simulink model "EcoSIM3_P2_C2_WIP"  (R2014b)
settings: Solver=ode1  SolverMode=SingleTasking  StartTime=0.0  StopTime=inf  FixedStep=0.01  RelTol=1e-3
PostLoadFcn:
  | %, if any(exist('dsrtsu_mdlpostloadfcn', 'file') == [2, 3, 6]), try dsrtsu_mdlpostloadfcn('Execute', bdroot); catch fprintf('Error in PostLoadFcn (dsrtsu_mdlpostloadfcn) for model "%s":\n %s\n', bdroot, lasterr); end, end,
InitFcn:
  | tic
  | %Startup_EcoSIM
values from neighbouring files (symbols this model uses):
  EngPwr = [0 5	10	15	20	25	30	35	40	45	50	55	60	65	70	75	80	85	90	95	100	105	110	115]    [Series_Maps.m]
  EngSpd = [0 477.4645 954.929 1909.858 2864.787 3819.716 4774.645 5729.574 6684.503]    [Series_Maps.m]
  EngTrq = [0	0	0	0	0	0	0	0	0	0	0	0	0	0	0	0	0	0	0	0	0	0	0	0 ... (first row only)    [Series_Maps.m]
  Power = [0 5 10 15 20 25 30]    [Series_Maps.m]
  Torque = [-50,-40,-30,-25,-20,-15,-10,-8,-6,-4,-2,0]    [Series_Maps.m]
undefined symbols (not defined in the file or in its folder): canChannel, Controls, DriveCycles, Driver, EM_EFF_MAP, EM_PwrLoss_MAP, Glbl, Overwritten_Mode, Plants, sigbuilder_block, Trialmap, Veh_Dynamics
libraries: simulink x141, canmsglib x113, fl_lib x104, canlib x89, nesl_utility x56, sdl_lib x29, dspsigops x6, dspswit3 x5, dspstat3 x2, commnoisgen2 x1, dspfdesign x1
(part 20 of 21)

== stateflow chart EcoSIM3_P2_C2_WIP/Powertrain/Electric Motor /Soft ECU/Algorithm/Startup_Shutdown/Startup-Shutdown ==
  state StartupShutdownSequence [group]
    state StartState
      entry: VSM_Mode = 0;
      during: Commanded_Torque = 0;
      %Loading EEPROM Parameters & carrying out POST (Power On Self Tests)
    state Standby
      % Entry point into Inverter
      % State Machine
    state Startup_Sequence
      state Inverter_Wait
        entry: VSM_Mode = 4;
        during: VSM_Mode = 4;
        during: Commanded_Torque =0;
        % Precharge_Bypasseed_EEPROM = 1
      state ReadyState
        entry: VSM_Mode = 5;
        during: VSM_Mode = 5;
        during: Commanded_Torque =0;
        en, du: Inverter_Enable_Lockout = 0;
      state MotorRunningState
        entry: Inverter_Enable_Lockout = 0;
        entry: Inverter_Status=1;
        during: Inverter_Enable_Lockout = 0;
      state MotorOnCommand
        entry: VSM_Mode=6;
      Inverter_Wait -> ReadyState : [KeySwMode == 0 && ...
          | Power_up==1]
      MotorOnCommand -> ReadyState [order 3] : [Inverter_Enable==0]
      ReadyState -> MotorRunningState : after(0.05,sec)
      MotorRunningState -> MotorOnCommand : [InternalMotorError==0 && Inverter_Enable == 1]
    state ShutdownInProcess
      entry: VSM_Mode = 14;
      entry: Inverter_Enable_Lockout=1;
      entry: Inverter_Status=0;
      during: VSM_Mode = 14;
    state FaultState
      entry: VSM_Mode = 7;
      during: VSM_Mode = 7;
    (junction 28) -> Standby [order 2]
    Standby -> StartState : [Power_up == 1]
    (default) -> (junction 28)
    ShutdownInProcess -> Standby : [KeySwMode == 0 && ...
        | Power_up == 0]
    StartState -> FaultState [order 2] : [POST_Fault == 1]
    StartState -> Inverter_Wait [order 1] : [Power_up ==1 && ...
        | ~InternalMotorError && POST_Fault == 0 ...
        | && batt_mainc_stat == 1 ]
    (junction 28) -> FaultState [order 1] : [InternalMotorError ==1]
    FaultState -> ShutdownInProcess : [(KeySwMode == 0 && ...
        | Power_up == 0) ]
    MotorOnCommand -> ShutdownInProcess [order 1] : [ShutdownRequest ==1]
    MotorOnCommand -> FaultState [order 2] : [RUN_Fault==1]
  data: Power_up input; VSM_Mode output; InternalMotorError input; batt_mainc_stat input; Inverter_Enable input; Inverter_Enable_Lockout output; RUN_Fault input; Commanded_Torque local; ShutdownRequest input; KeySwMode input; POST_Fault input; Inverter_Status output

== stateflow chart EcoSIM3_P2_C2_WIP/Powertrain/Electric Motor /Soft ECU/Algorithm/Normal Operation/Normal_Operation ==
  state NormalOperation
    entry: set_direction=Rotation_Direction;
    entry: ShutdownRequest=0;
    exit: Commanded_Torque=0;
    state SpeedGreaterThanMaxSpeed
      entry: Commanded_Torque=0;
    state ValidSpeed
      entry: Commanded_Torque=Torque_Command;
      during: Commanded_Torque=Torque_Command;
    (default) -> (junction 9)
    (junction 9) -> SpeedGreaterThanMaxSpeed [order 1] : [abs (Motor_Speed) > Motor_MaxSpeed]
    (junction 9) -> (junction 10) [order 2]
    SpeedGreaterThanMaxSpeed -> (junction 10) : [abs (Motor_Speed) <= Motor_MaxSpeed]
    (junction 10) -> ValidSpeed
    ValidSpeed -> SpeedGreaterThanMaxSpeed : [abs (Motor_Speed) > Motor_MaxSpeed]
  state Fault
    entry: RUN_Fault=1;
  state ShutdownRequest
    entry: ShutdownRequest=1;
  (default) -> NormalOperation
  NormalOperation -> Fault [order 1] : [ InternalMotorError ==1||batt_mainc_stat==0]
  NormalOperation -> ShutdownRequest [order 2] : [Power_up==0]
  ShutdownRequest -> NormalOperation : [Power_up==1]
  data: Motor_Speed input; InternalMotorError input; Rotation_Direction input; set_direction local; Commanded_Torque output; Torque_Command input; batt_mainc_stat input; Inverter_Enable input; Power_up input; RUN_Fault output; Motor_MaxSpeed input; ShutdownRequest output

== stateflow chart EcoSIM3_P2_C2_WIP/GCM/ProcessMode/Chart ==
  state Entry
    entry: charge_mode_request=0;
    Relay_Charge=0;
    Relay_Vehicle=0;
  state FaultMode
  state VehicleRunMode
    entry: charge_mode_request=0;
    Relay_Charge=1;
    Relay_Vehicle=1;
  state ChargingMode
    entry: charge_mode_request=1;
    Relay_Charge=1;
    Relay_Vehicle=0;
  (default) -> Entry
  VehicleRunMode -> Entry : [Key_State==0]
  ChargingMode -> Entry [order 1] : [GCM_Wakeup_charge==0]
  Entry -> VehicleRunMode [order 1] : [Key_State==1 && ...
      | GCM_Wakeup_charge==0]
  Entry -> FaultMode [order 3] : [Key_State==1 && ...
      | GCM_Wakeup_charge ==1]
  Entry -> ChargingMode [order 2] : [Key_State ==0 && ...
      | GCM_Wakeup_charge==1]
  ChargingMode -> FaultMode [order 2] : [Key_State==1]
  data: Key_State input; GCM_Wakeup_charge input; Relay_Charge output; Relay_Vehicle output; charge_mode_request output

== matlab function EcoSIM3_P2_C2_WIP/Supervisory Controller/Functional Safety1/Functional Safety Algorithm/Fault Management/Truth Table ==
  data: u input; y output
function y = fcn(u)

aVarTruthTableCondition_1 = false;
aVarTruthTableCondition_2 = false;


% Example condition 1

aVarTruthTableCondition_1 = logical(u >= 0);

% Example condition 2

aVarTruthTableCondition_2 = logical(u ^ 2 <= 1);

if (aVarTruthTableCondition_1 && aVarTruthTableCondition_2)
    aFcnTruthTableAction_1();
elseif (~aVarTruthTableCondition_1 && ~aVarTruthTableCondition_2)
    aFcnTruthTableAction_1();
else % Default
    aFcnTruthTableAction_2();
end

function aFcnTruthTableAction_1()

% Example action 1 called from D1 & D2 column in condition table

y = u;

function aFcnTruthTableAction_2()

% Example action 2 called from D3 column in condition table

y = 1 / u;

== stateflow chart EcoSIM3_P2_C2_WIP/Powertrain/Clutch_Transmission1/CP1 SoftEcu/Algorithm/Chart ==
  note: Clutch_Sw - 0= Clutch fully engaged
      |                        1= Clutch fully disengaged (Pedal completely pressed
      |                        2= Engagement/ Disengagement in process (This state has been introduced so that Mastershift does not shift
      | accidentally while clutch is being engaged, and GCM does not allow torque transmission before clutch is fully engaged
      |
      | Clutch_Request- Request to press (disengage) the clutch
      | 0= Engage the clutch  (Foot off the pedal)
      | 1= Disengage the clutch (Press the pedal)
  state Default
  state DisengageClutch
    entry: Clutch_Engage=0;
    entry: Clutch_Sw=2;
    during: Clutch_Sw=2;
  state ClutchDisengaged
    entry: Clutch_Engage=0;
    entry:Clutch_Sw=1;
  state EngageClutch
    entry: Clutch_Engage=1;
    entry: Clutch_Sw=2;
    during: Clutch_Sw=2;
  state ClutchEngaged
    entry: Clutch_Engage=1;
    entry:Clutch_Sw=0;
    during:Clutch_Sw=0;
  (default) -> Default
  Default -> EngageClutch [order 2] : [Clutch_Request==0]
  Default -> DisengageClutch [order 1] : [Clutch_Request==1]
  ClutchEngaged -> DisengageClutch : [Clutch_Request==1]
  DisengageClutch -> ClutchDisengaged [order 2] : [Clutch_Pressure<=5]
  EngageClutch -> DisengageClutch [order 2] : [Clutch_Request==1]
  DisengageClutch -> EngageClutch [order 1] : [Clutch_Request==0]
  ClutchDisengaged -> EngageClutch : [Clutch_Request==0]
  EngageClutch -> ClutchEngaged [order 1] : [Clutch_Pressure>=10]
  data: Clutch_Request input; Clutch_Pressure input; Clutch_Engage output; Clutch_Sw output

== stateflow chart EcoSIM3_P2_C2_WIP/Supervisory Controller/Mode Operation/Limited EV/Temperature Limiting Old/Chart ==
  state EM
    entry: out=1
  state Normal
    entry: out=4;
  state Inverter
    entry: out=2
  state Battery
    entry: out=3
  Normal -> EM [order 1] : [EM>100]
  (default) -> Normal
  Normal -> Inverter [order 2] : [Inverter>70]
  Normal -> Battery [order 3] : [Battery>50]
  data: EM input; Inverter input; Battery input; out output

== stateflow chart EcoSIM3_P2_C2_WIP/Fault Insertion/ESS Triggers/Chart ==
  state init
    en: output = 40;
  state stage1
    en: output = 56;
  state stage2
    en: output = 66;
  state stage3
    en: output = 40;
  (default) -> init
  init -> stage1 : [in == 1]
  stage1 -> stage2 : after(20, sec)
  stage2 -> stage3 : after(20, sec)
  data: in input; output output

== stateflow chart EcoSIM3_P2_C2_WIP/Supervisory Controller/Mode Operation/Series1/Engine Torque Request ==
  state Entry
    entry: Torque_Request=0;
  state TorqueRequest
    state FullTorque
      entry: Torque_Request= 100-2*(BAS_Speed-Desired_BAS_Speed);
      during: Torque_Request= 100-2*(BAS_Speed-Desired_BAS_Speed);
    state FullTorque1
      entry: Torque_Request= 100;
    FullTorque1 -> FullTorque : [BAS_Speed>Desired_BAS_Speed]
    FullTorque -> FullTorque1 : [BAS_Speed<Desired_BAS_Speed]
    (default) -> FullTorque1
  (default) -> Entry
  TorqueRequest -> Entry : [BAS_Speed>Desired_BAS_Speed+10]
  Entry -> TorqueRequest : [BAS_Speed<410]
  data: BAS_Speed input; Torque_Request output; Desired_BAS_Speed input

== stateflow chart EcoSIM3_P2_C2_WIP/Supervisory Controller/Charging Handshake/Chart1 ==
  state Entry
    entry: chga_wake=0;
    PON=0;
    Charging_Complete=0;
  state ChargeRequest
    entry: chga_wake=1;
  state ChargeComplete
    entry: PON=0;
    en: chga_wake=0;
    en: Charging_Complete=1;
  state OktoCharge
    entry: PON=1;
  note: Enable the DCDC and start cooling fans here
  (default) -> Entry
  OktoCharge -> Entry [order 2] : [charge_mode_request==0]
  ChargeRequest -> Entry [order 2] : [charge_mode_request==0]
  Entry -> ChargeRequest : [charge_mode_request==1]
  ChargeRequest -> OktoCharge [order 1] : [chga_ena==1 && bcm_ready==1 && ...
      | bcm_on_plug==1]
  OktoCharge -> ChargeComplete [order 1] : [bcm_chg_done==1 && ...
      | bcm_balancing==0]
  data: charge_mode_request input; chga_ena input; chga_wake output; PON output; bcm_chg_done input; bcm_balancing input; Charging_Complete output; bcm_ready input; bcm_on_plug input

== stateflow chart EcoSIM3_P2_C2_WIP/Supervisory Controller/Mode Operation/Shutdown/Shutdown/ESS Handshake ==
  note: The ESS handshake ensures that the hsc_bcm_enable signal commands is sent by the supervisory only when the bcm is in the appropriate readiness state
  state WaitforBCMReady1
  state Disable
    entry: hsc_bcm_enable=0;
    during: hsc_bcm_enable=0;
  state OpenContactors
    entry:hsc_bcm_mainc_close=0;
    entry: hsc_bcm_leakage_ena=1;
    during:hsc_bcm_mainc_close=0;
    during:hsc_bcm_enable=0;
  Disable -> WaitforBCMReady1 : [bcm_ready==0]
  OpenContactors -> Disable : [bcm_mainc_stat==0]
  (default) -> OpenContactors
  data: bcm_ready input double; bcm_cpwr_cmd input double; bcm_cpwr_mon input double; hsc_bcm_enable output double; hsc_bcm_mainc_close output double; hsc_bcm_leakage_ena output; bcm_veh_mon input; Veh_Start input double; bcm_mainc_stat input

== stateflow chart EcoSIM3_P2_C2_WIP/Supervisory Controller/PRNDL/Park/Check EM Limits/Chart ==
  state Entry
    en, du: Inverter_Enable=0;
    en, du: Torque_Command=0;
  state ChangeDirection
    en, du: Rotation_Direction=0;
    en, du: Torque_Command=0;
  state EnableInverter
    en, du: Inverter_Enable=1;
    en, du: Torque_Command=0;
  state TransmitTorque
    entry: Torque_Command=0;
    during: Torque_Command=0;
  (default) -> Entry
  TransmitTorque -> Entry : [Direction_Command_Feedback~=0 || ...
      | Inverter_Enable_Lockout==1]
  EnableInverter -> Entry [order 2] : [Inverter_Enable_Lockout==1]
  Entry -> ChangeDirection
  ChangeDirection -> EnableInverter : [Inverter_Enable_Lockout==0&& ...
      | Enable_Request==1]
  EnableInverter -> TransmitTorque [order 1] : [VSM_State==6&& ...
      | Direction_Command_Feedback==0]
  data: Enable_Request input; Torque_Request input; Inverter_Enable_Lockout input; VSM_State input; Direction_Command_Feedback input; Inverter_Enable output; Rotation_Direction output; Torque_Command output

== stateflow chart EcoSIM3_P2_C2_WIP/Supervisory Controller/Mode Operation/Startup/BAS Start up/BAS Handshake ==
  state Entry
    entry: BAS_Mode_Request=0;
  state EnableBASInverter
    entry: BAS_Mode_Request=1;
  (default) -> Entry
  Entry -> EnableBASInverter : [BAS_Fault_Status==0 ...
      | && bcm_mainc_stat==1]
  data: BAS_Fault_Status input; bcm_mainc_stat input; BAS_Mode_Request output

== stateflow chart EcoSIM3_P2_C2_WIP/Supervisory Controller/Mode Operation/Startup/Battery Start Up /ESS Handshake ==
  note: The ESS handshake ensures that the hsc_bcm_enable signal commands is sent by the supervisory only when the bcm is in the appropriate readiness state
  state Entry
    entry: hsc_bcm_enable=0;
    en: hsc_bcm_leakage_ena=1;
    en: hsc_bcm_mainc_close=0;
  state WaitforBCMReady
  state Enable
    entry: hsc_bcm_enable=1;
    during: hsc_bcm_enable=1;
  state CloseContactors
    entry:hsc_bcm_mainc_close=1;
    during:hsc_bcm_mainc_close=1;
    during:hsc_bcm_enable=1;
  (default) -> Entry
  Entry -> WaitforBCMReady : [bcm_veh_mon==1 && Veh_Start==1]
  WaitforBCMReady -> Enable : [bcm_ready==1]
  Enable -> CloseContactors : [bcm_cpwr_cmd==1 && bcm_cpwr_mon==1]
  data: bcm_ready input double; bcm_cpwr_cmd input double; bcm_cpwr_mon input double; hsc_bcm_enable output double; hsc_bcm_mainc_close output double; hsc_bcm_leakage_ena output; bcm_veh_mon input; bcm_mainc_stat input; Veh_Start input double

== stateflow chart EcoSIM3_P2_C2_WIP/Supervisory Controller/Mode Operation/Startup/EM Start up/EM Handshake ==
  state DisableInverter
    entry: Inverter_Enable=0;
    during: Inverter_Enable=0;
  state EnableInverter
    entry: Inverter_Enable=1;
    during: Inverter_Enable=1;
  (default) -> DisableInverter
  EnableInverter -> DisableInverter : [Inverter_Enable_Lockout==1]
  DisableInverter -> EnableInverter : [Inverter_Enable_Lockout==0 ...
      | && bcm_mainc_stat==1 ...
      | && SysPwrMd==2]
  data: bcm_mainc_stat input; Inverter_Enable_Lockout input; Inverter_Enable output; SysPwrMd input

== stateflow chart EcoSIM3_P2_C2_WIP/Supervisory Controller/Mode Operation/Startup/Vehicle Ready ==
  state Entry
    entry: Vehicle_Ready=0;
  state Started
    entry:Vehicle_Ready=1;
  (default) -> Entry
  Entry -> Started : [bcm_mainc_stat==1 ...
      | && Inverter_Enable ==1 ...
      | && BAS_Mode_Request ==1 ...
      | &&Startup_Complete==1]
  data: Startup_Complete input; bcm_mainc_stat input; Inverter_Enable input; BAS_Mode_Request input; Vehicle_Ready output

== stateflow chart EcoSIM3_P2_C2_WIP/Supervisory Controller/PRNDL/Reverse/Check EM Limits/Chart ==
  state Entry
    en, du: Inverter_Enable=0;
    en, du: Torque_Command=0;
    State=0;
  state ChangeDirection
    en, du: Rotation_Direction=1;
    en, du: Torque_Command=0;
    State=1;
  state EnableInverter
    en, du: Inverter_Enable=1;
    en, du: Torque_Command=0;
    State=2;
  state TransmitTorque
    entry: Torque_Command=Torque_Request;
    during: Torque_Command=Torque_Request;
    State=3;
  (default) -> Entry
  EnableInverter -> Entry [order 2] : [Inverter_Enable_Lockout==1]
  TransmitTorque -> Entry : [Direction_Command_Feedback~=1 || ...
      | Inverter_Enable_Lockout==1]
  Entry -> ChangeDirection
  ChangeDirection -> EnableInverter : [Inverter_Enable_Lockout==0&& ...
      | Enable_Request==1]
  EnableInverter -> TransmitTorque [order 1] : [VSM_State==6&& ...
      | Direction_Command_Feedback==1]
  data: Enable_Request input; Torque_Request input; Inverter_Enable_Lockout input; VSM_State input; Direction_Command_Feedback input; Inverter_Enable output; Rotation_Direction output; Torque_Command output; State output

== stateflow chart EcoSIM3_P2_C2_WIP/Supervisory Controller/PRNDL/Neutral /Check EM Limits/Chart ==
  state Entry
    en, du: Inverter_Enable=0;
    en, du: Torque_Command=0;
  state ChangeDirection
    en, du: Rotation_Direction=0;
    en, du: Torque_Command=0;
  state EnableInverter
    en, du: Inverter_Enable=1;
    en, du: Torque_Command=0;
  state TransmitTorque
    entry: Torque_Command=Torque_Request;
    during: Torque_Command=Torque_Request;
  (default) -> Entry
  EnableInverter -> Entry [order 2] : [Inverter_Enable_Lockout==1]
  TransmitTorque -> Entry : [Direction_Command_Feedback~=0 || ...
      | Inverter_Enable_Lockout==1]
  Entry -> ChangeDirection
  ChangeDirection -> EnableInverter : [Inverter_Enable_Lockout==0&& ...
      | Enable_Request==1]
  EnableInverter -> TransmitTorque [order 1] : [VSM_State==6 && ...
      | Direction_Command_Feedback==0]
  data: Enable_Request input; Torque_Request input; Inverter_Enable_Lockout input; VSM_State input; Direction_Command_Feedback input; Inverter_Enable output; Rotation_Direction output; Torque_Command output

== stateflow chart EcoSIM3_P2_C2_WIP/Supervisory Controller/PRNDL/Drive/Check EM Limits/Chart ==
  state Entry
    en, du: Inverter_Enable=0;
    en, du: Torque_Command=0;
  state ChangeDirection
    en, du: Rotation_Direction=0;
    en, du: Torque_Command=0;
  state EnableInverter
    en, du: Inverter_Enable=1;
    en, du: Torque_Command=0;
  state TransmitTorque
    entry: Torque_Command=Torque_Request;
    during: Torque_Command=Torque_Request;
  (default) -> Entry
  TransmitTorque -> Entry : [Direction_Command_Feedback~=0 || ...
      | Inverter_Enable_Lockout==1]
  EnableInverter -> Entry [order 2] : [Inverter_Enable_Lockout==1]
  Entry -> ChangeDirection
  ChangeDirection -> EnableInverter : [Inverter_Enable_Lockout==0&& ...
      | Enable_Request==1]
  EnableInverter -> TransmitTorque [order 1] : [VSM_State==6 && ...
      | Direction_Command_Feedback==0]
  data: Enable_Request input; Torque_Request input; Inverter_Enable_Lockout input; VSM_State input; Direction_Command_Feedback input; Inverter_Enable output; Rotation_Direction output; Torque_Command output

== stateflow chart EcoSIM3_P2_C2_WIP/Powertrain/Clutch_Transmission1/GCM/GCM Soft ECU/Shift Signal Generator ==
  note: Clutch-Transmission Soft ECU
      | When the softECU receives a gear change request and a torque rampdown complete flag from the supervisory
      | it asks for the clutch to be disengaged. It reports TCU gear as 0 and does not allow torque rampup. It then commands
      | shift from current gear to neutral, and then from neutral to the desired gear. It then asks for clutch engagement,  reports
      | updated gear to supervisory, and allows torque rampup
  note: Can we use TCM_Gear for comparison everywhere
      | and get rid of Actual_Gear?
  state Default
    entry: Bypasscount=0;
    Clutch_Request=0;
  note: We do not need to put a clutch condition here
      | as it will be given to Mastershift
  state ShiftState
    entry: Local_Count=0;
    entry:Shift_Count= Local_Gear_Request - Actual_Gear;
  state NoShift
    entry: Clutch_Request=0;
  note: Second last bypass put in
      | Shift_Count at 0.
      | Bad logic.
      | Find better.
  state StartPressin
    entry: Local_Gear_Request=Gear_Request;
  note: Do we have clutch request before the
      | upshift/ downshift blips or after them?
      | Mastershift shoud be fine either ways.
      | It might change the time we set to count
      | the blips by the soft ecu
  state UpshiftRequest
    entry: Upshift_Sw=1;
    en: Local_Count = Local_Count + 1;
  state DownshiftRequest
    entry: Downshift_Sw=1;
    en: Local_Count = Local_Count + 1;
  note: Blip generator
  state ClutchRelease
    entry: Clutch_Request=0;
  state Wait1
  state Wait2
  state Wait3
  state Wait4
  state WaitState
    entry: Upshift_Sw=0;
  state WaitState1
    entry: Downshift_Sw=0;
  state Wait
  state Bypasscounter
    entry: Bypasscount = Bypasscount + 1;
  state ClutchRequest
    entry: Upshift_Sw=0;
    entry: Downshift_Sw=0;
    entry: Clutch_Request=1;
  note: Most recent bypass
  (default) -> Default
  Default -> NoShift
  StartPressin -> ShiftState
  Bypasscounter -> NoShift
  ClutchRelease -> NoShift
  ShiftState -> UpshiftRequest [order 1] : [Shift_Count > 0]
  ShiftState -> Wait [order 3] : [Shift_Count==0]
  ShiftState -> DownshiftRequest [order 2] : [Shift_Count < 0]
  NoShift -> StartPressin : [Gear_Request~=Actual_Gear]
  UpshiftRequest -> Wait1 [order 1] : [abs(Shift_Count)~=Local_Count]
  Wait2 -> UpshiftRequest : after (0.01,sec)
  UpshiftRequest -> Wait [order 2] : [abs(Shift_Count)==Local_Count]
  DownshiftRequest -> Wait [order 2] : [abs(Shift_Count)==Local_Count]
  DownshiftRequest -> Wait3 [order 1] : [abs(Shift_Count)~=Local_Count]
  Wait4 -> DownshiftRequest : after (0.01,sec)
  Wait1 -> WaitState : after(0.01, sec)
  WaitState -> Wait2
  Wait3 -> WaitState1 : after(0.01,sec)
  WaitState1 -> Wait4
  ClutchRequest -> ClutchRelease [order 1] : [Actual_Gear==Local_Gear_Request]
  Wait -> ClutchRequest : after(0.01, sec)
  ClutchRequest -> Bypasscounter [order 2] : after (3,sec)
  data: Clutch_Request output; Gear_Request input; Local_Gear_Request local; Local_Count local; Shift_Count local; Upshift_Sw output; Downshift_Sw output; Actual_Gear input; Bypasscount local

== stateflow chart EcoSIM3_P2_C2_WIP/Powertrain/Clutch_Transmission1/Mastershift Softecu/Algorithm/Chart ==
  note: Do we implement the clutch timeout as given in Mastershift doc?
      | We won't need it because supervisory will always give clutch request
      | along with gear request
  state ResetCounter
    entry: reset=-5;
  note: Time period taken into consideration to count the
      | no. of Upshifts/ Downshifts
  state Comeon
    entry: reset=0;
    entry: Local_Count=Count;
    entry: Gear_Cmd=Actual_Gear;
    entry: TCM_Gear=Actual_Gear;
  state Start
    entry: Local_Count=Count;
    entry:reset=0;
    during: Local_Count=Count;
  state CounterReset
    entry: reset=1;
  state StartShifting
    entry: Gear_Cmd=Actual_Gear+round(Local_Count);
    entry: TCM_Gear=0;
    during: Gear_Cmd=Actual_Gear+round(Local_Count);
  note: Currently, the softecu directly receives the Gear requested by the GCM and proceeds to shift into that gear when
      | the clutch is pressed.
      | The final softecu is supposed to receive 'Upshift' and 'Downshift' commands from the GCM in the form of blips.
      | It will then count the number of blips and add it to the existing gear, effectively counting the gear requested.
      | The timeout state is set so that if the softecu does not receive confirmation that the clutch is disengaged some time
      | after the gear change request is received, it will not shift. The timeout values are generally between (3000 ms and 5000 ms)
      | according the Mastershift documentation. We probably won't require the timeout function in the softecu because the GCM
      | should take care of the clutch command.
      | This stateflow now loops between Default and Timeout Wait if the ClutchSw~=1 and Gear Requested is kept the same. The
      | cancelling of the original gear request can be implemented using the reset counter once the Upshift/Downshift is completed
  state ShiftingComplete
    entry: TCM_Gear=Actual_Gear;
    entry: reset=-5; %Counter has rising edge trigger
    during: TCM_Gear=Actual_Gear;
    during: Local_Count=Count;
  ResetCounter -> Start
  StartShifting -> ResetCounter [order 2] : [Gear_Cmd>5||Gear_Cmd<1]
  (default) -> Comeon
  Start -> CounterReset : [Clutch_Sw==1]
  Comeon -> Start : [Count~=0]
  CounterReset -> StartShifting
  ShiftingComplete -> Comeon : [Clutch_Sw==0]
  StartShifting -> ShiftingComplete [order 1] : [Actual_Gear==Gear_Cmd]
  data: Clutch_Sw input; Actual_Gear input; Gear_Cmd output; TCM_Gear output; reset output; Local_Count local; Count input

== stateflow chart EcoSIM3_P2_C2_WIP/Supervisory Controller/Mode Selection /Limp Home Mode Selection  /Chart ==
  state Engine_Only
    entry: VEH_Mode=3;
  state EV_Limited
    entry: VEH_Mode=5;
  state Normal_Operation
    entry: VEH_Mode=2;
  state Shutdown
    entry: VEH_Mode=6;
  Normal_Operation -> Engine_Only [order 1] : [Fault_Code==1]
  Engine_Only -> Shutdown : [Fault_Code==3]
  Normal_Operation -> EV_Limited [order 2] : [Fault_Code==2]
  EV_Limited -> Shutdown : [Fault_Code==3]
  Normal_Operation -> Shutdown [order 3] : [Fault_Code==3]
  (default) -> (junction 7)
  (junction 7) -> Normal_Operation : [Fault_Code==0]
  data: VEH_Mode output; Fault_Code input

== stateflow chart EcoSIM3_P2_C2_WIP/Supervisory Controller/Mode Selection /Mode Selection  ==
  state Vehicle_On
    state Series
      entry: VEH_Mode=9;
    state CD_Normal
      entry: VEH_Mode=2;
    state Engine_on
      entry: VEH_Mode=3;
    state Engine_Start
      entry: VEH_Mode=4;
    Engine_on -> CD_Normal : [eng_switch==0&&SOC<Min_SOC]
    Series -> CD_Normal : [cs_switch==0||SOC>95]
    Engine_Start -> Series [order 1] : [eng_on==1&&...
        | cs_switch==1]
    (default) -> CD_Normal
    Engine_Start -> Engine_on [order 2] : [eng_on==1&&...
        | eng_switch==1]
    CD_Normal -> Engine_Start : [SOC<Min_SOC || eng_switch==1||...
        | cs_switch==1]
  state Startup
    entry: VEH_Mode=1;
  state Accessory
    entry: VEH_Mode=7;
  state Shutdown
    entry: VEH_Mode=6;
  state Charging
    entry: VEH_Mode=8;
  (default) -> Startup
  Startup -> Vehicle_On [order 1] : [SysPwrMd==2&&Vehicle_Ready>0]
  Startup -> Charging [order 3] : [bcm_on_plug==1]
  Shutdown -> Startup : [Shutdown_Complete==1&&SysPwrMd>0]
  Startup -> Accessory [order 2] : [SysPwrMd==1]
  Vehicle_On -> Accessory [order 2] : [SysPwrMd==1]
  Vehicle_On -> Charging [order 3] : [bcm_on_plug==1]
  Vehicle_On -> Shutdown [order 1] : [SysPwrMd==0]
  Accessory -> Shutdown : [SysPwrMd==0]
  Charging -> Shutdown : [bcm_on_plug==0]
  data: Veh_Spd input; SOC input; VEH_Mode output; Min_SOC input; beta input; SysPwrMd input; eng_on input; eng_switch input; cs_switch input; Vehicle_Ready input; Shutdown_Complete input; bcm_on_plug input

== matlab function EcoSIM3_P2_C2_WIP/Supervisory Controller/PRNDL/Determine Gear/Truth Table ==
  data: y output; PRNDL input double; Force_Neutral input boolean; Force_Park input boolean
function y = fcn(PRNDL, Force_Neutral, Force_Park)

aVarTruthTableCondition_1 = false;
aVarTruthTableCondition_2 = false;
aVarTruthTableCondition_3 = false;
aVarTruthTableCondition_4 = false;
aVarTruthTableCondition_5 = false;
aVarTruthTableCondition_6 = false;


% Force Park

aVarTruthTableCondition_1 = logical(Force_Park == 1);

% Force Neutral

aVarTruthTableCondition_2 = logical(Force_Neutral == 1);

% PRNDL set to P

aVarTruthTableCondition_3 = logical(PRNDL == 1);

% PRNDL set to R

aVarTruthTableCondition_4 = logical(PRNDL == 2);

% PRNDL set to N

aVarTruthTableCondition_5 = logical(PRNDL == 3);

% PRNDL set to D

aVarTruthTableCondition_6 = logical(PRNDL == 4);

if (aVarTruthTableCondition_1)
    aFcnTruthTableAction_1();
elseif (aVarTruthTableCondition_2)
    aFcnTruthTableAction_3();
elseif (aVarTruthTableCondition_3)
    aFcnTruthTableAction_1();
elseif (~aVarTruthTableCondition_1 && ~aVarTruthTableCondition_2 && ~aVarTruthTableCondition_3 && aVarTruthTableCondition_4 && ~aVarTruthTableCondition_5 && ~aVarTruthTableCondition_6)
    aFcnTruthTableAction_2();
elseif (~aVarTruthTableCondition_1 && ~aVarTruthTableCondition_3 && ~aVarTruthTableCondition_4 && aVarTruthTableCondition_5 && ~aVarTruthTableCondition_6)
    aFcnTruthTableAction_3();
elseif (~aVarTruthTableCondition_1 && ~aVarTruthTableCondition_2 && ~aVarTruthTableCondition_3 && ~aVarTruthTableCondition_4 && ~aVarTruthTableCondition_5 && aVarTruthTableCondition_6)
    aFcnTruthTableAction_4();
else % Default
    aFcnTruthTableAction_1();
end

function aFcnTruthTableAction_1()

% Vehicle is in PARK gear

y = 1;

function aFcnTruthTableAction_2()

% Vehicle is in REVERSE gear

y = 2;

function aFcnTruthTableAction_3()

% Vehicle is in NEUTRAL gear

y = 3;

function aFcnTruthTableAction_4()

% Vehicle is in DRIVE gear

y = 4;

== matlab function EcoSIM3_P2_C2_WIP/Supervisory Controller/Input Conditioning/PRNDL Conditioning/Truth Table ==
  data: u input; PRNDL1 output; PRNDL2 output double; PRNDL3 output double
function [PRNDL1, PRNDL2, PRNDL3] = fcn(u)

aVarTruthTableCondition_1 = false;
aVarTruthTableCondition_2 = false;
aVarTruthTableCondition_3 = false;
aVarTruthTableCondition_4 = false;


% Park

aVarTruthTableCondition_1 = logical(u == 1);

% Reverse

aVarTruthTableCondition_2 = logical(u == 2);

% Neutral

aVarTruthTableCondition_3 = logical(u == 3);

% Drive

aVarTruthTableCondition_4 = logical(u == 4);

if (aVarTruthTableCondition_1 && ~aVarTruthTableCondition_2 && ~aVarTruthTableCondition_3 && ~aVarTruthTableCondition_4)
    aFcnTruthTableAction_1();
elseif (~aVarTruthTableCondition_1 && aVarTruthTableCondition_2 && ~aVarTruthTableCondition_3 && ~aVarTruthTableCondition_4)
    aFcnTruthTableAction_2();
elseif (~aVarTruthTableCondition_1 && ~aVarTruthTableCondition_2 && aVarTruthTableCondition_3 && ~aVarTruthTableCondition_4)
    aFcnTruthTableAction_3();
elseif (~aVarTruthTableCondition_1 && ~aVarTruthTableCondition_2 && ~aVarTruthTableCondition_3 && aVarTruthTableCondition_4)
    aFcnTruthTableAction_4();
else % Default
    aFcnTruthTableAction_5();
end

function aFcnTruthTableAction_1()

% Park

PRNDL1 = 1; PRNDL2=15; PRNDL3=0;

function aFcnTruthTableAction_2()

% Reverse

PRNDL1 = 2; PRNDL2=14; PRNDL3=2;

function aFcnTruthTableAction_3()

% Neutral

PRNDL1 = 3; PRNDL2=13; PRNDL3=0;

function aFcnTruthTableAction_4()

% Drive

PRNDL1 = 4; PRNDL2=13; PRNDL3=1;

function aFcnTruthTableAction_5()

% Between Ranges

PRNDL1 = 0; PRNDL2=0; PRNDL3=3;

== stateflow chart EcoSIM3_P2_C2_WIP/Supervisory Controller/Mode Operation/Startup/BAS_Signals/BAS Handshake ==
  state Entry
    entry: BAS_Mode_Request=0;
  state EnableBASInverter
    entry: BAS_Mode_Request=1;
  (default) -> Entry
  Entry -> EnableBASInverter : [BAS_Fault_Status==0 ...
      | && bcm_mainc_stat==1]
  data: BAS_Fault_Status input; bcm_mainc_stat input; BAS_Mode_Request output

== stateflow chart EcoSIM3_P2_C2_WIP/Supervisory Controller/Mode Operation/Engine Only /Trans Clutch Messages/GentleClutchRelease ==
  state Entry
    entry: Shift_Request=0;
  state EngagementTransition
    entry: Shift_Request=0;
    exit: Shift_Request=0;
    state LowSpeed
      entry: Shift_Request=0;
    state Transition
      entry: Shift_Request=1.5*(BAS_Speed-Lower_Clutch_Speed);
      during: Shift_Request=1.5*(BAS_Speed-Lower_Clutch_Speed);
    state FullyEngaged
      entry: Shift_Request=100;
    (default) -> LowSpeed
    Transition -> LowSpeed [order 1] : [BAS_Speed<=Lower_Clutch_Speed]
    FullyEngaged -> LowSpeed [order 1] : [BAS_Speed<=Lower_Clutch_Speed]
    LowSpeed -> Transition : [BAS_Speed>Lower_Clutch_Speed+5]
    Transition -> FullyEngaged [order 2] : [BAS_Speed>=Upper_Clutch_Speed+5]
    FullyEngaged -> Transition [order 2] : [BAS_Speed<Upper_Clutch_Speed]
  (default) -> Entry
  EngagementTransition -> Entry : [Clutch_Request==0]
  Entry -> EngagementTransition : [Clutch_Request==1]
  data: BAS_Speed input; Clutch_Request input; Lower_Clutch_Speed input; Upper_Clutch_Speed input; Shift_Request output

== matlab function EcoSIM3_P2_C2_WIP/Supervisory Controller/PRNDL/Determine Gear1/Truth Table ==
  data: y output; PRNDL input double; Force_Neutral input boolean
function y = fcn(PRNDL, Force_Neutral)

aVarTruthTableCondition_1 = false;
aVarTruthTableCondition_2 = false;
aVarTruthTableCondition_3 = false;
aVarTruthTableCondition_4 = false;
aVarTruthTableCondition_5 = false;
aVarTruthTableCondition_6 = false;


% Force Neutral

aVarTruthTableCondition_1 = logical(Force_Neutral == 1);

% PRNDL invalid gear

aVarTruthTableCondition_2 = logical(PRNDL == 0);

% PRNDL set to P

aVarTruthTableCondition_3 = logical(PRNDL == 1);

% PRNDL set to R

aVarTruthTableCondition_4 = logical(PRNDL == 2);

% PRNDL set to N

aVarTruthTableCondition_5 = logical(PRNDL == 3);

% PRNDL set to D

aVarTruthTableCondition_6 = logical(PRNDL == 4);

if (aVarTruthTableCondition_1)
    aFcnTruthTableAction_3();
elseif (aVarTruthTableCondition_2)
    aFcnTruthTableAction_3();
elseif (~aVarTruthTableCondition_1 && ~aVarTruthTableCondition_2 && ~aVarTruthTableCondition_3 && aVarTruthTableCondition_4 && ~aVarTruthTableCondition_5 && ~aVarTruthTableCondition_6)
    aFcnTruthTableAction_2();
elseif (~aVarTruthTableCondition_1 && ~aVarTruthTableCondition_2 && ~aVarTruthTableCondition_3 && ~aVarTruthTableCondition_4 && ~aVarTruthTableCondition_5 && aVarTruthTableCondition_6)
    aFcnTruthTableAction_1();
else % Default
    aFcnTruthTableAction_3();
end

function aFcnTruthTableAction_1()

% Vehicle is in FORWARD gear

y = 1;

function aFcnTruthTableAction_2()

% Vehicle is in REVERSE gear

y = 2;

function aFcnTruthTableAction_3()

% Vehicle is in NEUTRAL gear

y = 3;

== stateflow chart EcoSIM3_P2_C2_WIP/Powertrain/Engine/Soft ECU/Algorithm/TorqueRegulation/Subsystem/Chart ==
  state Entry
    en, du: Torque_Cmd=0;
    Mode = 1;
  state PoweredUp
    en, du: Torque_Cmd=0;
    Mode = 1;
  state Normal_Operation
    state Idling
      en, du: Mode = 2;
      state IdlingTorque [commented out]
        entry: Torque_Cmd =25;
      state NoTorque [commented out]
        entry: Torque_Cmd=0;
      NoTorque -> IdlingTorque [commented out] : [Engine_Speed <...
          | Lower_Idle_Speed_Bound]
      IdlingTorque -> NoTorque [commented out] : [Engine_Speed>...
          | Upper_Idle_Speed_Bound]
      (default) -> NoTorque [commented out]
    state Operational
      en, du: Torque_Cmd=Torque_Request;
      Torque_Cmd=Torque_Request;
      Mode = 3;
    state Engine_Overspeed
      en, du: Torque_Cmd=0;
      Mode = 4;
    (default) -> (junction 33)
    (junction 33) -> Idling [order 2]
    (junction 33) -> Operational [order 1] : [Engine_Speed >Lower_Idle_Speed_Bound]
    Operational -> Idling [order 2] : [Engine_Speed <Lower_Idle_Speed_Bound]
    Idling -> Operational : [Torque_Request >10&&...
        | Engine_Speed>Upper_Idle_Speed_Bound]
    Operational -> Engine_Overspeed [order 1] : [Engine_Speed>Max_Speed]
    Engine_Overspeed -> Operational : [Engine_Speed <(Max_Speed-15)]
  (default) -> Entry
  Normal_Operation -> Entry [order 1] : [ECM_Powerup==0]
  Entry -> PoweredUp : [ECM_Powerup==1]
  Normal_Operation -> PoweredUp [order 2] : [PCM_Wake==0 || ...
      | ISP_R ==0]
  PoweredUp -> Normal_Operation : [PCM_Wake==1 &&...
      | ISP_R==1]
  data: Engine_Speed input; ECM_Powerup input; Torque_Cmd output; Torque_Request input; PCM_Wake input; ISP_R input; Max_Speed input; Upper_Idle_Speed_Bound input; Lower_Idle_Speed_Bound input; Mode output

== stateflow chart EcoSIM3_P2_C2_WIP/Supervisory Controller/Clutch Request/GCM Request ==
  state Entry
    entry: Clutch_Request=0;
    GCM_Gear_Request=Actual_Gear;
    Shift_In_Progress=0;
  state SetLocalGear
    entry: GCM_Gear_Request=Gear_Request;
    Clutch_Request=1;
    Shift_In_Progress=1;
  state ShiftComplete
    entry:Clutch_Request=0;
    Shift_In_Progress=0;
  (default) -> Entry
  Entry -> SetLocalGear : [Gear_Request~=Actual_Gear]
  ShiftComplete -> SetLocalGear : [Gear_Request~=Actual_Gear]
  SetLocalGear -> ShiftComplete : [Shift_Complete==1]
  data: Actual_Gear input; Shift_Complete input; Gear_Request input; GCM_Gear_Request output; Clutch_Request output; Shift_In_Progress output

== stateflow chart EcoSIM3_P2_C2_WIP/GCM/ProcessMode/MastershiftMessages/Shift Signal Generator ==
  note: Clutch-Transmission Soft ECU
      | When the softECU receives a gear change request and a torque rampdown complete flag from the supervisory
      | it asks for the clutch to be disengaged. It reports TCU gear as 0 and does not allow torque rampup. It then commands
      | shift from current gear to neutral, and then from neutral to the desired gear. It then asks for clutch engagement,  reports
      | updated gear to supervisory, and allows torque rampup
  note: Can we use TCM_Gear for comparison everywhere
      | and get rid of Actual_Gear?
  note: We do not need to put a clutch condition here
      | as it will be given to Mastershift
  state Default
    entry: Bypasscount=0;
    Clutch_Sw=0;
    Shift_Complete=1;
  state ShiftState
    entry: Local_Count=0;
    state=2;
    entry:Shift_Count= GCM_Gear_Request - Gear_From_Mastershift;
    Shift_Complete=0;
  state NoShift
    entry: Clutch_Sw=0;
    Shift_Complete=1;
    state=1;
    exit: Shift_Complete=0;
  note: Second last bypass put in
      | Shift_Count at 0.
      | Bad logic.
      | Find better.
  note: Do we have clutch request before the
      | upshift/ downshift blips or after them?
      | Mastershift shoud be fine either ways.
      | It might change the time we set to count
      | the blips by the soft ecu
  state UpshiftRequest
    entry: Upshift_Sw=1;
    en: Local_Count = Local_Count + 1;
  state DownshiftRequest
    entry: Downshift_Sw=1;
    en: Local_Count = Local_Count + 1;
    state=3;
  note: Blip generator
  state ClutchRelease
    entry: Shift_Complete=1;
    state=5;
  state Wait1
  state Wait2
  state Wait3
  state Wait4
  note: Add a timeout on state ClutchRelease
      | to take care of Clutch riding and subsequent
      | downshift
  state WaitState
    entry: Upshift_Sw=0;
  state WaitState1
    entry: Downshift_Sw=0;
  state Wait
  state WaitForClutchDisengaged
    entry: Upshift_Sw=0;
    entry: Downshift_Sw=0;
    Shift_Count=0;
    Local_Count=0;
    state=4;
  state ClutchRequest
    entry: Upshift_Sw=0;
    entry: Downshift_Sw=0;
    entry: Clutch_Sw=1;
  state Bypasscounter
    entry: Bypasscount = Bypasscount + 1;
  note: Most recent bypass
  (default) -> Default
  Default -> NoShift
  Bypasscounter -> ShiftState
  NoShift -> ShiftState : [GCM_Gear_Request~=Gear_From_Mastershift]
  ShiftState -> UpshiftRequest [order 2] : [Shift_Count > 0]
  ShiftState -> Wait [order 1] : [Shift_Count==0]
  ShiftState -> DownshiftRequest [order 3] : [Shift_Count < 0]
  ClutchRelease -> NoShift
  UpshiftRequest -> Wait1 [order 1] : [abs(Shift_Count)~=Local_Count]
  Wait2 -> UpshiftRequest : after (0.01,sec)
  UpshiftRequest -> Wait [order 2] : [abs(Shift_Count)==Local_Count]
  DownshiftRequest -> Wait [order 2] : [abs(Shift_Count)==Local_Count]
  DownshiftRequest -> Wait3 [order 1] : [abs(Shift_Count)~=Local_Count]
  Wait4 -> DownshiftRequest : after (0.01,sec)
  Wait1 -> WaitState : after(0.01, sec)
  WaitState -> Wait2
  Wait3 -> WaitState1 : after(0.01,sec)
  WaitState1 -> Wait4
  ClutchRequest -> ClutchRelease [order 1] : [Gear_From_Mastershift==GCM_Gear_Request]
  Wait -> WaitForClutchDisengaged : after(0.01, sec)
  WaitForClutchDisengaged -> ClutchRequest : [Clutch_Status==1]
  ClutchRequest -> Bypasscounter [order 2] : after (3,sec)
  data: GCM_Gear_Request input; Clutch_Status input; Upshift_Sw output; Downshift_Sw output; Gear_From_Mastershift input; Bypasscount local; Clutch_Sw output; Local_Count output; Shift_Count output; state output; Shift_Complete output

== stateflow chart EcoSIM3_P2_C2_WIP/Supervisory Controller/Mode Operation/Engine Only /TM Messages/EM Torque Request ==
  state Default
    entry: Torque_Request=0;
  state Torque
    entry: Torque_Request=0.2*Driver_Request;
    during:Torque_Request=0.2*Driver_Request;
  (default) -> Default
  Default -> Torque : [Alpha>90]
  Torque -> Default : [Alpha<85]
  data: Driver_Request input; Alpha input; Torque_Request output

== stateflow chart EcoSIM3_P2_C2_WIP/Powertrain/Clutch_Transmission2/Trans_Plant/Plant/Subsystem/Determine Gear ==
  state NotNeutral
    state FifthReverse
      state DetermineGear3
      state First
        entry: Gear=5;
      state Second
        entry: Gear=-1;
      (default) -> DetermineGear3
      DetermineGear3 -> NotNeutral.FifthReverse.Second [order 1] : [y5R==3]
      DetermineGear3 -> NotNeutral.FifthReverse.First [order 2] : [y5R==1]
      NotNeutral.FifthReverse.First -> NotNeutral.FifthReverse.Second : [y5R==3]
      NotNeutral.FifthReverse.Second -> NotNeutral.FifthReverse.First : [y5R==1]
    state ThirdFourth
      state DetermineGear2
      state First
        entry: Gear=3;
      state Second
        entry: Gear=4;
      (default) -> DetermineGear2
      DetermineGear2 -> NotNeutral.ThirdFourth.First [order 2] : [y34==1]
      DetermineGear2 -> NotNeutral.ThirdFourth.Second [order 1] : [y34==3]
      NotNeutral.ThirdFourth.First -> NotNeutral.ThirdFourth.Second : [y34==3]
      NotNeutral.ThirdFourth.Second -> NotNeutral.ThirdFourth.First : [y34==1]
    state FirstSecond
      state DetermineGear1
      state First
        entry: Gear=1;
      state Second
        entry: Gear=2;
      (default) -> DetermineGear1
      DetermineGear1 -> NotNeutral.FirstSecond.First [order 2] : [y12==1]
      DetermineGear1 -> NotNeutral.FirstSecond.Second [order 1] : [y12==3]
      NotNeutral.FirstSecond.First -> NotNeutral.FirstSecond.Second : [y12==3]
      NotNeutral.FirstSecond.Second -> NotNeutral.FirstSecond.First : [y12==1]
    state DetermineGear
    DetermineGear -> FirstSecond [order 1] : [y12~=2 && ...
        | y34==2 && ...
        | y5R==2]
    FirstSecond -> DetermineGear : [y12==2]
    DetermineGear -> FifthReverse [order 3] : [y12==2 && ...
        | y34==2 && ...
        | y5R ~=2]
    FifthReverse -> DetermineGear : [y5R==2]
    DetermineGear -> ThirdFourth [order 2] : [y12==2 && ...
        | y34~=2 && ...
        | y5R==2]
    ThirdFourth -> DetermineGear : [y34==2]
    (default) -> DetermineGear
  state Neutral
    entry: Gear=0;
  (default) -> Neutral
  Neutral -> NotNeutral : [y12~=2 || ...
      | y34~=2 || ...
      | y5R~=2]
  NotNeutral -> Neutral : [y12==2 && ...
      | y34==2 &&...
      | y5R==2]
  data: y12 input; y34 input; y5R input; Gear output

== matlab function EcoSIM3_P2_C2_WIP/Powertrain/Clutch_Transmission2/Trans_Plant/Plant/Subsystem/Truth Table ==
  data: u1 input; y output; u2 input double; u3 input double
function y = fcn(u1, u2, u3)

aVarTruthTableCondition_1 = false;
aVarTruthTableCondition_2 = false;
aVarTruthTableCondition_3 = false;
aVarTruthTableCondition_4 = false;
aVarTruthTableCondition_5 = false;
aVarTruthTableCondition_6 = false;
aVarTruthTableCondition_7 = false;
aVarTruthTableCondition_8 = false;
aVarTruthTableCondition_9 = false;


% 12

aVarTruthTableCondition_1 = logical(u1==2);

% 22

aVarTruthTableCondition_2 = logical(u2==2);

% 32

aVarTruthTableCondition_3 = logical(u3==2);

% 11

aVarTruthTableCondition_4 = logical(u1==1);

% 13

aVarTruthTableCondition_5 = logical(u1==3);

% 21

aVarTruthTableCondition_6 = logical(u2==1);

% 23

aVarTruthTableCondition_7 = logical(u2==3);

% 31

aVarTruthTableCondition_8 = logical(u3==1);

% 33

aVarTruthTableCondition_9 = logical(u3==3);

if (aVarTruthTableCondition_1 && aVarTruthTableCondition_2 && aVarTruthTableCondition_3 && ~aVarTruthTableCondition_4 && ~aVarTruthTableCondition_5 && ~aVarTruthTableCondition_6 && ~aVarTruthTableCondition_7 && ~aVarTruthTableCondition_8 && ~aVarTruthTableCondition_9)
    aFcnTruthTableAction_1();
elseif (~aVarTruthTableCondition_1 && aVarTruthTableCondition_2 && aVarTruthTableCondition_3 && aVarTruthTableCondition_4 && ~aVarTruthTableCondition_5 && ~aVarTruthTableCondition_6 && ~aVarTruthTableCondition_7 && ~aVarTruthTableCondition_8 && ~aVarTruthTableCondition_9)
    aFcnTruthTableAction_2();
elseif (~aVarTruthTableCondition_1 && aVarTruthTableCondition_2 && aVarTruthTableCondition_3 && ~aVarTruthTableCondition_4 && aVarTruthTableCondition_5 && ~aVarTruthTableCondition_6 && ~aVarTruthTableCondition_7 && ~aVarTruthTableCondition_8 && ~aVarTruthTableCondition_9)
    aFcnTruthTableAction_3();
elseif (aVarTruthTableCondition_1 && ~aVarTruthTableCondition_2 && aVarTruthTableCondition_3 && ~aVarTruthTableCondition_4 && ~aVarTruthTableCondition_5 && aVarTruthTableCondition_6 && ~aVarTruthTableCondition_7 && ~aVarTruthTableCondition_8 && ~aVarTruthTableCondition_9)
    aFcnTruthTableAction_4();
elseif (aVarTruthTableCondition_1 && ~aVarTruthTableCondition_2 && aVarTruthTableCondition_3 && ~aVarTruthTableCondition_4 && ~aVarTruthTableCondition_5 && ~aVarTruthTableCondition_6 && aVarTruthTableCondition_7 && ~aVarTruthTableCondition_8 && ~aVarTruthTableCondition_9)
    aFcnTruthTableAction_5();
elseif (aVarTruthTableCondition_1 && aVarTruthTableCondition_2 && ~aVarTruthTableCondition_3 && ~aVarTruthTableCondition_4 && ~aVarTruthTableCondition_5 && ~aVarTruthTableCondition_6 && ~aVarTruthTableCondition_7 && aVarTruthTableCondition_8 && ~aVarTruthTableCondition_9)
    aFcnTruthTableAction_6();
elseif (aVarTruthTableCondition_1 && aVarTruthTableCondition_2 && ~aVarTruthTableCondition_3 && ~aVarTruthTableCondition_4 && ~aVarTruthTableCondition_5 && ~aVarTruthTableCondition_6 && ~aVarTruthTableCondition_7 && ~aVarTruthTableCondition_8 && aVarTruthTableCondition_9)
    aFcnTruthTableAction_7();
else % Default
    aFcnTruthTableAction_8();
end

function aFcnTruthTableAction_1()

% Neutral

y=0;

function aFcnTruthTableAction_2()

% First

y=1;

function aFcnTruthTableAction_3()

% Second

y=2;

function aFcnTruthTableAction_4()

% Third

y=3;

function aFcnTruthTableAction_5()

% Fourth

y=4;

function aFcnTruthTableAction_6()

% Fifth

y=5;

function aFcnTruthTableAction_7()

% Reverse

y=-1;

function aFcnTruthTableAction_8()

% Invalid

y=8;

== matlab function EcoSIM3_P2_C2_WIP/Powertrain/Clutch_Transmission2/Trans_Plant/Plant/Truth Table ==
  data: y3 output double; u input; y2 output double; y1 output
function [y3, y2, y1] = fcn(u)

aVarTruthTableCondition_1 = false;
aVarTruthTableCondition_2 = false;
aVarTruthTableCondition_3 = false;
aVarTruthTableCondition_4 = false;
aVarTruthTableCondition_5 = false;
aVarTruthTableCondition_6 = false;
aVarTruthTableCondition_7 = false;


% Gear 1

aVarTruthTableCondition_1 = logical(u==1);

% Gear 2

aVarTruthTableCondition_2 = logical(u==2);

% Gear 3

aVarTruthTableCondition_3 = logical(u==3);

% Gear 4

aVarTruthTableCondition_4 = logical(u==4);

% Gear 5

aVarTruthTableCondition_5 = logical(u==5);

% Gear N

aVarTruthTableCondition_6 = logical(u==0);

% Gear R

aVarTruthTableCondition_7 = logical(u==-1);

if (aVarTruthTableCondition_1 && ~aVarTruthTableCondition_2 && ~aVarTruthTableCondition_3 && ~aVarTruthTableCondition_4 && ~aVarTruthTableCondition_5 && ~aVarTruthTableCondition_6 && ~aVarTruthTableCondition_7)
    aFcnTruthTableAction_1();
elseif (~aVarTruthTableCondition_1 && aVarTruthTableCondition_2 && ~aVarTruthTableCondition_3 && ~aVarTruthTableCondition_4 && ~aVarTruthTableCondition_5 && ~aVarTruthTableCondition_6 && ~aVarTruthTableCondition_7)
    aFcnTruthTableAction_2();
elseif (~aVarTruthTableCondition_1 && ~aVarTruthTableCondition_2 && aVarTruthTableCondition_3 && ~aVarTruthTableCondition_4 && ~aVarTruthTableCondition_5 && ~aVarTruthTableCondition_6 && ~aVarTruthTableCondition_7)
    aFcnTruthTableAction_3();
elseif (~aVarTruthTableCondition_1 && ~aVarTruthTableCondition_2 && ~aVarTruthTableCondition_3 && aVarTruthTableCondition_4 && ~aVarTruthTableCondition_5 && ~aVarTruthTableCondition_6 && ~aVarTruthTableCondition_7)
    aFcnTruthTableAction_4();
elseif (~aVarTruthTableCondition_1 && ~aVarTruthTableCondition_2 && ~aVarTruthTableCondition_3 && ~aVarTruthTableCondition_4 && aVarTruthTableCondition_5 && ~aVarTruthTableCondition_6 && ~aVarTruthTableCondition_7)
    aFcnTruthTableAction_5();
elseif (~aVarTruthTableCondition_1 && ~aVarTruthTableCondition_2 && ~aVarTruthTableCondition_3 && ~aVarTruthTableCondition_4 && ~aVarTruthTableCondition_5 && aVarTruthTableCondition_6 && ~aVarTruthTableCondition_7)
    aFcnTruthTableAction_6();
elseif (~aVarTruthTableCondition_1 && ~aVarTruthTableCondition_2 && ~aVarTruthTableCondition_3 && ~aVarTruthTableCondition_4 && ~aVarTruthTableCondition_5 && ~aVarTruthTableCondition_6 && aVarTruthTableCondition_7)
    aFcnTruthTableAction_7();
else % Default
    aFcnTruthTableAction_6();
end

function aFcnTruthTableAction_1()

% Gear 1

y1=-16;
y2=0;
y3=0;

function aFcnTruthTableAction_2()

% Gear 2

y1=16;
y2=0;
y3=0;

function aFcnTruthTableAction_3()

% Gear 3

y1=0;
y2=-16;
y3=0;

function aFcnTruthTableAction_4()

% Gear 4

y1=0;
y2=16;
y3=0;

function aFcnTruthTableAction_5()

% Gear 5

y1=0;
y2=0;
y3=-16;

function aFcnTruthTableAction_6()

% Neutral

y1=0;
y2=0;
y3=0;

function aFcnTruthTableAction_7()

% Reverse

y1=0;
y2=0;
y3=16;

== stateflow chart EcoSIM3_P2_C2_WIP/Supervisory Controller/Simple Fault Detection/Fault Code Determination ==
  state Normal_Operation
    entry: Fault_Code=0;
  state Limited_EV
    entry: Fault_Code=2;
  state Shutdown
    entry: Fault_Code=3;
  Limited_EV -> Normal_Operation [order 2] : [EM_Temp<EM_Warning-3&&...
      | Inverter_Temp<Inverter_Warning-3&&...
      | bcm_dis_buf>=90]
  Normal_Operation -> Limited_EV [order 1] : [EM_Temp>EM_Warning&&EM_Temp<EM_Shutdown||...
      | Inverter_Temp>Inverter_Warning&&Inverter_Temp<Inverter_Shutdown||...
      | bcm_dis_buf<85&&Battery_Temp<Battery_Shutdown]
  (default) -> Normal_Operation
  Limited_EV -> Shutdown [order 1] : [EM_Temp>=EM_Shutdown||...
      | Inverter_Temp>=Inverter_Shutdown||...
      | Battery_Temp>=Battery_Shutdown...
      | || bcm_dis_buf<=10]
  Normal_Operation -> Shutdown [order 2] : [EM_Temp>=EM_Shutdown||...
      | Inverter_Temp>=Inverter_Shutdown||...
      | Battery_Temp>=Battery_Shutdown||...
      | bcm_dis_buf<=10]
  data: EM_Temp input; Battery_Temp input; Inverter_Temp input; Fault_Code output; EM_Warning input; EM_Shutdown input; Inverter_Warning input; Inverter_Shutdown input; bcm_dis_buf input; Battery_Shutdown input
